simulink model "bh_slopey_floor_rolling_sphere_MASK"  (R2020b)
settings: Solver=ode15s  StartTime=0.0  StopTime=6  FixedStep=0.001  RelTol=1e-6  EnableMultiTasking=on
undefined symbols (not defined in the file): X, Y, Z
libraries: nesl_utility x25, sm_lib x21
settings Model: EnablePacing=on  Creator=scastro  LastModifiedBy=bhorton
settings SolverCC: ZeroCrossAlgorithm=Adaptive
settings DataIOCC: LimitDataPoints=on  ReturnWorkspaceOutputs=off
settings OptimizationCC: BlockReduction=off  LifeSpan=inf
settings DebuggingCC: AllowSymbolicDim=off  SFUnexpectedBacktrackingDiag=warning  SFNoUnconditionalDefaultTransitionDiag=warning  SFExecutionAtInitializationDiag=none  ArithmeticOperatorsInVariantConditions=warning
settings SFSimCC: SimUseLocalCustomCode=off  CustomCodeUndefinedFunction=UseInterfaceOnly
settings RTWCC: RTWUseLocalCustomCode=off
settings CodeAppCC: StateflowObjectComments=on
settings GRTTargetCC: TargetLangStandard=C89/C90 (ANSI)
settings ConfigComp: CovMetricSettings=dw  CovSaveCumulativeToWorkspaceVar=on  CovSaveSingleToWorkspaceVar=on  CovExternalEMLEnable=off  CovSFcnEnable=off
settings SimscapeCC: SimscapeNormalizeSystem=off  SimscapeLogType=all  SimscapeLogLimitData=off  SimscapeLogDataHistory=10000
settings ConfigurationSet: Description=SimMechanics 2G
settings DiagnosticsConfigSet: SimMechanicsRigidlyBoundBlock=none
settings ExplorerConfigSet: InternalSimMechanicsExplorerSettings="<ExplorerConfiguration><canonicalview>default</canonicalview><AnimationSetting><BasePlaybackSpeed>1.0</BasePlaybackSpeed><PlaybackSpeedFactor>1.0</PlaybackSpeedFactor></AnimationSetting><TilePanel><TileInfo><Tiles Columns=\"2\" Count=\"4\" Rows=\"2\"><Column Weight=\"0.4996\"/><Column Weight=\"0.5004\"/><Row Weight=\"0.4994\"/><Row Weight=\"0.5006\"/><Tile Height=\"1\" Width=\"1\" X=\"0\" Y=\"0\"/><Tile Height=\"1\" Width=\"1\" X=\"0\" Y=\"1\"/><Tile Height=\"1\" Width=\"1\" X=\"1\" Y=\"0\"/><Tile Height=\"1\" Width=\"1\" X=\"1\" Y=\"1\"/></Tiles></TileInfo><SceneInfo><SceneViewer><BGColor><R>0.60000002384185791</R><G>0.60000002384185791</G><B>0.60000002384185791</B></BGColor><Camera><DoPerspective>off</DoPerspective><Position><X>2.25966727667424827</X><Y>-62.0130897867078019</Y><Z>-2.35818613645341157</Z></Position><Center><X>2.25966727667424827</X><Y>-2.62125395139589656e-07</Y><Z>-2.35818613645341157</Z></Center><Up><X>0</X><Y>-0</Y><Z>1</Z></Up><ViewLimDist>1</ViewLimDist><YLim>12.1061815480941526</YLim><XLim>17.886610575562532</XLim></Camera></SceneViewer><SceneViewer><BGColor><R>0.60000002384185791</R><G>0.60000002384185791</G><B>0.60000002384185791</B></BGColor><Camera><DoPerspective>off</DoPerspective><Position><X>13.7336956207032639</X><Y>-7.76347886559767453</Y><Z>61.1905876504773261</Z></Position><Center><X>13.7336956207032639</X><Y>-7.76347886559767453</Y><Z>-0.181522868139726512</Z></Center><Up><X>0</X><Y>1</Y><Z>-0</Z></Up><ViewLimDist>1</ViewLimDist><YLim>19.5392058706914682</YLim><XLim>28.7392803837973183</XLim></Camera></SceneViewer><SceneViewer><BGColor><R>0.60000002384185791</R><G>0.60000002384185791</G><B>0.60000002384185791</B></BGColor><Camera><DoPerspective>off</DoPerspective><Position><X>62.80059271421446</X><Y>5.74913462249758478</Y><Z>-9.58222127968170945</Z></Position><Center><X>1.37359199311038616</X><Y>5.74913462249758478</Y><Z>-9.58222127968170945</Z></Center><Up><X>-0</X><Y>0</Y><Z>1</Z></Up><ViewLimDist>1</ViewLimDist><YLim>22.3277388712980738</YLim><XLim>33.0893067056624588</XLim></Camera></SceneViewer><SceneViewer><BGColor><R>0.60000002384185791</R><G>0.60000002384185791</G><B>0.60000002384185791</B></BGColor><Camera><DoPerspective>off</DoPerspective><Position><X>61.5862213655142483</X><Y>-21.6336600450757075</Y><Z>3.54423065630081169</Z></Position><Center><X>22.1204892369751072</X><Y>14.8464342674815555</Y><Z>-10.516698059065412</Z></Center><Up><X>-0.213092164247365046</X><Y>0.142054424815019287</Y><Z>0.9666500245315508</Z></Up><ViewLimDist>1</ViewLimDist><YLim>31.0369134821928654</YLim><XLim>45.7898858100513593</XLim></Camera></SceneViewer></SceneInfo></TilePanel><MechEditorPanel><Cameras/><GfxPanelCameraMap/><VideoCreator><PlaybackSpeedRatio>1.0</PlaybackSpeedRatio><FrameRate>30</FrameRate><VideoFormat>Motion JPEG AVI</VideoFormat><FrameSize>auto</FrameSize></VideoCreator></MechEditorPanel></ExplorerConfiguration>"

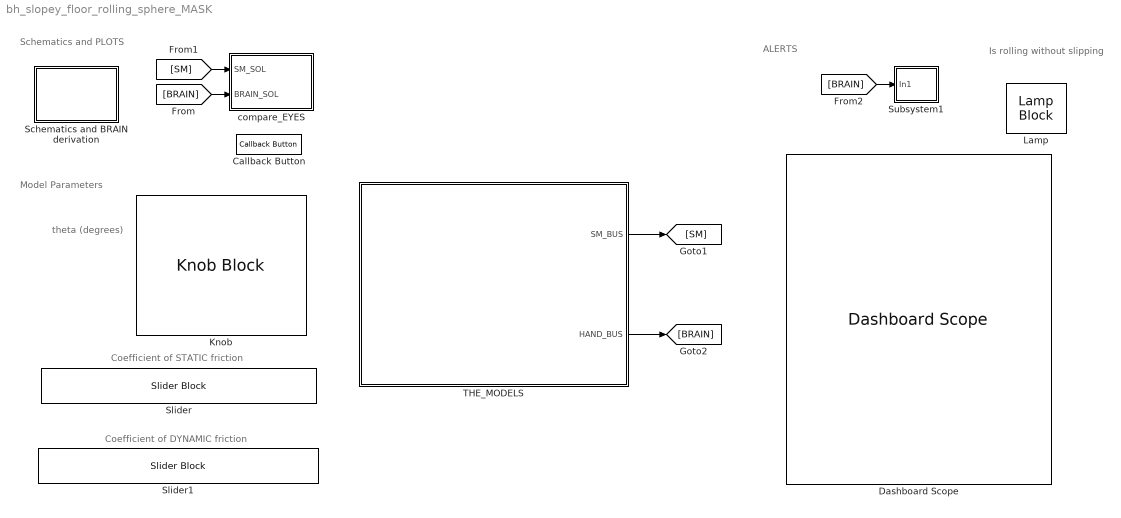
== system bh_slopey_floor_rolling_sphere_MASK ==
  note: Is rolling without slipping
  note: ALERTS
  note: theta (degrees)
  note: Model Parameters
  note: Schematics and PLOTS
  note: Coefficient of DYNAMIC friction
  note: Coefficient of STATIC friction
  Callback Button : CallbackButton  ButtonText=OPEN scope
      settings: ClickFcn="open_system(bdroot+\"/compare_EYES/compare_scope\")"
  Dashboard Scope : DashboardScope
  Knob : KnobBlock  LabelPosition=Hide  ScaleMin=5  ScaleMax=75  TickInterval=5
  Lamp : LampBlock
  Schematics and BRAIN derivation : Subsystem
  Slider : SliderBlock  LabelPosition=Hide  ScaleMax=0.5  TickInterval=0.05
  Slider1 : SliderBlock  LabelPosition=Hide  ScaleMax=0.3  TickInterval=0.05
  Subsystem1 : Subsystem
  THE_MODELS : Subsystem  mask{sphRad=1.5, sphMass=1, theta_deg=30, mu_static=0.5, mu_dynamic=0.3, g=9.80665}
      mask prompts: sphRad "Radius  (m)"; sphMass "Mass (kg)"; theta_deg "theta  (DEGREES)"; mu_static "Coefficient of STATIC friction"; mu_dynamic "Coefficient of DYNAMIC friction"; g "g  (m/sec^2)"
      mask DialogControl Container4 Prompt: Sphere
      mask DialogControl Container5 Prompt: Floor
      mask DialogControl Container6 Prompt: Friction
      mask DialogControl Container7 Prompt: Environment
      mask Display: image('bh_MASK_PIC_DO_NOT_DELETE.PNG'); % Use "Edit Image" on toolstrip to change.
  compare_EYES : Subsystem
  wires:
  [SM] -> compare_EYES/1(SM_SOL)
  [BRAIN] -> compare_EYES/2(BRAIN_SOL)
  THE_MODELS/1(SM_BUS) -> [SM]
  THE_MODELS/2(HAND_BUS) -> [BRAIN]
  [BRAIN] -> Subsystem1/1(In1)

== system bh_slopey_floor_rolling_sphere_MASK/Schematics and BRAIN derivation ==
  note: Open the BRAIN derivation
  note: Open the Simulink implementation of the BRAIN derivation
  Callback Button : CallbackButton  ButtonText=Open the BRAIN Derivation
      settings: ClickFcn=open bh_hand_deriv_sphere_on_slopey_floor.PDF
  Callback Button1 : CallbackButton  ButtonText=Open the Simulink Implementation
      settings: ClickFcn=|
      | THE_SYS = [bdroot,'/THE_MODELS/BRAIN_SOLUTION'];
      | open_system(THE_SYS)

== system bh_slopey_floor_rolling_sphere_MASK/Subsystem1 ==
  In1 : Inport
  Bus Selector : BusSelector  OutputSignals=tf_is_rolling,Ff_mag,N,muStat_times_N
  Terminator{,1..3} (4 alike) : Terminator
  wires:
  In1/1 -> Bus Selector/1
  Bus Selector/1 -> Terminator/1  "<tf_is_rolling>"
  Bus Selector/2 -> Terminator1/1  "<Ff_mag>"
  Bus Selector/3 -> Terminator2/1  "<N>"
  Bus Selector/4 -> Terminator3/1  "<muStat_times_N>"

== system bh_slopey_floor_rolling_sphere_MASK/THE_MODELS ==
  BRAIN_SOLUTION : Subsystem
  Simscape_Model : Subsystem
  SM_BUS : Outport
  HAND_BUS : Outport  Port=2
  wires:
  Simscape_Model/1(SM_BUS) -> SM_BUS/1
  BRAIN_SOLUTION/1(HAND_SOL) -> HAND_BUS/1

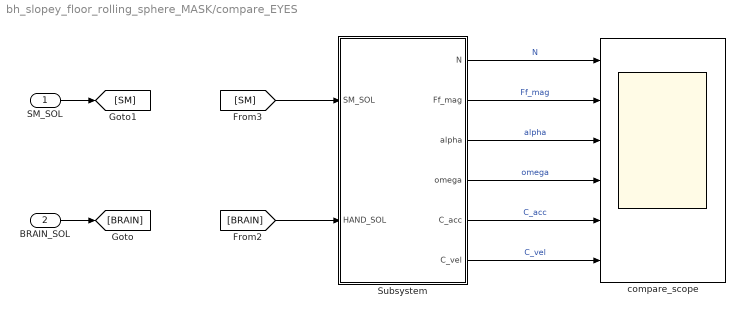
== system bh_slopey_floor_rolling_sphere_MASK/compare_EYES ==
  SM_SOL : Inport
  BRAIN_SOL : Inport  Port=2
  Subsystem : Subsystem
  compare_scope : Scope  NumInputPorts=6
  wires:
  BRAIN_SOL/1 -> [BRAIN]
  SM_SOL/1 -> [SM]
  [BRAIN] -> Subsystem/2(HAND_SOL)
  [SM] -> Subsystem/1(SM_SOL)
  Subsystem/1(N) -> compare_scope/1  "N"
  Subsystem/2(Ff_mag) -> compare_scope/2  "Ff_mag"
  Subsystem/3(alpha) -> compare_scope/3  "alpha"
  Subsystem/4(omega) -> compare_scope/4  "omega"
  Subsystem/5(C_acc) -> compare_scope/5  "C_acc"
  Subsystem/6(C_vel) -> compare_scope/6  "C_vel"

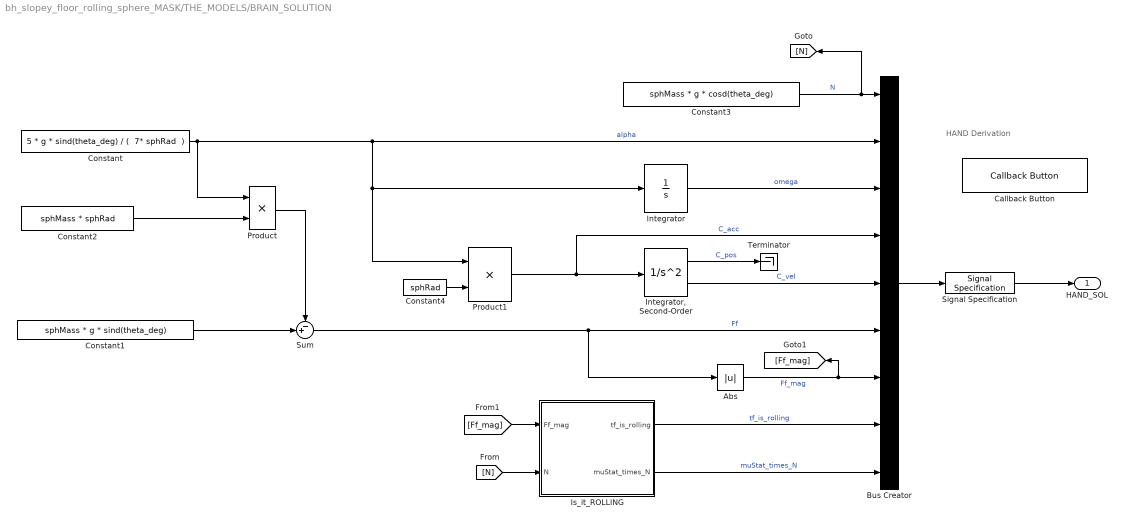
== system bh_slopey_floor_rolling_sphere_MASK/THE_MODELS/BRAIN_SOLUTION ==
  note: HAND Derivation
  Abs : Abs
  Bus Creator : BusCreator  Inputs=9
  Callback Button : CallbackButton  ButtonText=Open the hand Derivation
      settings: ClickFcn=open bh_hand_deriv_sphere_on_slopey_floor.PDF
  Constant : Constant  Value="5 * g * sind(theta_deg) / (  7* sphRad  )"
  Constant1 : Constant  Value=sphMass * g * sind(theta_deg)
  Constant2 : Constant  Value=sphMass * sphRad
  Constant3 : Constant  Value=sphMass * g * cosd(theta_deg)
  Constant4 : Constant  Value=sphRad
  Integrator : Integrator
  "Integrator, Second-Order" : SecondOrderIntegrator
  Is_it_ROLLING : Subsystem
  Product : Product
  Product1 : Product
  Signal Specification : SignalSpecification  SampleTime=0
  Sum : Sum  Inputs=-+|
  Terminator : Terminator
  HAND_SOL : Outport
  wires:
  Constant/1 -> Bus Creator/2, Integrator/1, Product1/1, Product/1  "alpha"
  Constant2/1 -> Product/2
  Product/1 -> Sum/1
  Constant1/1 -> Sum/2
  Constant3/1 -> [N], Bus Creator/1  "N"
  Sum/1 -> Abs/1, Bus Creator/6  "Ff"
  Abs/1 -> [Ff_mag], Bus Creator/7  "Ff_mag"
  Integrator/1 -> Bus Creator/3  "omega"
  Product1/1 -> "Integrator, Second-Order"/1, Bus Creator/4  "C_acc"
  Constant4/1 -> Product1/2
  "Integrator, Second-Order"/1 -> Terminator/1  "C_pos"
  "Integrator, Second-Order"/2 -> Bus Creator/5  "C_vel"
  Bus Creator/1 -> Signal Specification/1
  Signal Specification/1 -> HAND_SOL/1
  [Ff_mag] -> Is_it_ROLLING/1(Ff_mag)
  [N] -> Is_it_ROLLING/2(N)
  Is_it_ROLLING/1(tf_is_rolling) -> Bus Creator/8  "tf_is_rolling"
  Is_it_ROLLING/2(muStat_times_N) -> Bus Creator/9  "muStat_times_N"

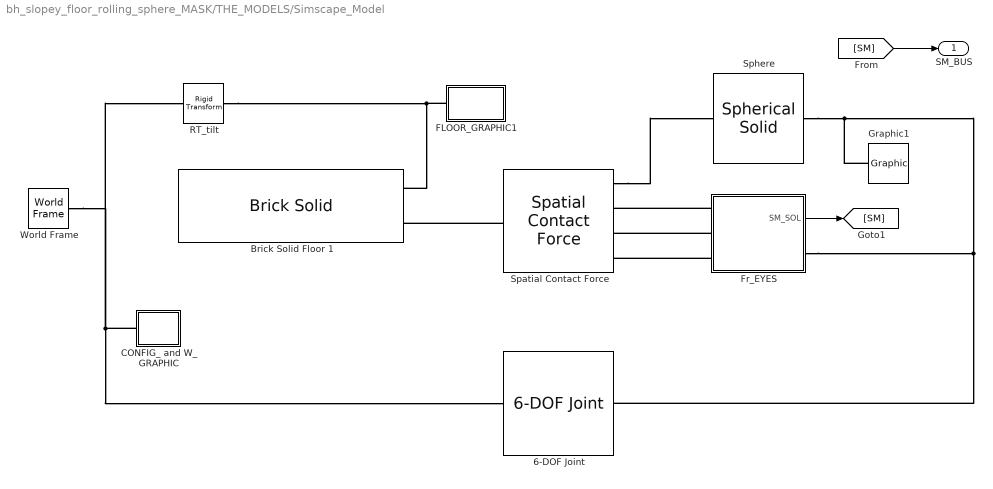
== system bh_slopey_floor_rolling_sphere_MASK/THE_MODELS/Simscape_Model ==
  6-DOF Joint : sm_lib/Joints/6-DOF Joint  JointMode=Normal  SenseConstraintForce=off  SenseConstraintForceX=off  SenseConstraintForceY=off  SenseConstraintForceZ=off  SenseConstraintTorque=off  SenseConstraintTorqueX=off  SenseConstraintTorqueY=off  SenseConstraintTorqueZ=off  SenseTotalForce=off  SenseTotalForceX=off  SenseTotalForceY=off  SenseTotalForceZ=off  SenseTotalTorque=off  SenseTotalTorqueX=off  SenseTotalTorqueY=off  SenseTotalTorqueZ=off  CompositeWrenchDir=FollowerOnBase  CompositeWrenchFrame=BaseFrame  PxEquilibriumPosition=0  PxEquilibriumPositionUnits=m  PxSpringStiffness=0  PxSpringStiffnessUnits=N/m  PxDampingCoefficient=0  PxDampingCoefficientUnits=N/(m/s)  PxTorqueActuationMode=NoTorque  PxMotionActuationMode=ComputedMotion  PxSensePosition=off  PxSenseVelocity=off  PxSenseAcceleration=off  PxSenseTorqueForce=off  PxSenseLowerLimitTorqueForce=off  PxSenseUpperLimitTorqueForce=off  PxLowerLimitSpecify=off  PxLowerLimitBound=-1  PxLowerLimitBoundUnits=m  PxLowerLimitStiffness=1e6  PxLowerLimitStiffnessUnits=N/m  PxLowerLimitDamping=1e3  PxLowerLimitDampingUnits=N/(m/s)  PxLowerLimitTransitionRegionWidth=1e-4  PxLowerLimitTransitionRegionWidthUnits=m  PxUpperLimitSpecify=off  PxUpperLimitBound=1  PxUpperLimitBoundUnits=m  PxUpperLimitStiffness=1e6  PxUpperLimitStiffnessUnits=N/m  PxUpperLimitDamping=1e3  PxUpperLimitDampingUnits=N/(m/s)  PxUpperLimitTransitionRegionWidth=1e-4  PxUpperLimitTransitionRegionWidthUnits=m  PxPositionTargetSpecify=on  PxPositionTargetPriority=High  PxPositionTargetValue=sphRad*sind(theta_deg)  PxPositionTargetValueUnits=m  PxVelocityTargetSpecify=off  PxVelocityTargetPriority=High  PxVelocityTargetValue=0  PxVelocityTargetValueUnits=m/s  PyEquilibriumPosition=0  PyEquilibriumPositionUnits=m  PySpringStiffness=0  PySpringStiffnessUnits=N/m  PyDampingCoefficient=0  PyDampingCoefficientUnits=N/(m/s)  PyTorqueActuationMode=NoTorque  PyMotionActuationMode=ComputedMotion  PySensePosition=off  PySenseVelocity=off  PySenseAcceleration=off  PySenseTorqueForce=off  PySenseLowerLimitTorqueForce=off  PySenseUpperLimitTorqueForce=off  PyLowerLimitSpecify=off  PyLowerLimitBound=-1  PyLowerLimitBoundUnits=m  PyLowerLimitStiffness=1e6  PyLowerLimitStiffnessUnits=N/m  PyLowerLimitDamping=1e3  PyLowerLimitDampingUnits=N/(m/s)  PyLowerLimitTransitionRegionWidth=1e-4  PyLowerLimitTransitionRegionWidthUnits=m  PyUpperLimitSpecify=off  PyUpperLimitBound=1  PyUpperLimitBoundUnits=m  PyUpperLimitStiffness=1e6  PyUpperLimitStiffnessUnits=N/m  PyUpperLimitDamping=1e3  PyUpperLimitDampingUnits=N/(m/s)  PyUpperLimitTransitionRegionWidth=1e-4  PyUpperLimitTransitionRegionWidthUnits=m  PyPositionTargetSpecify=on  PyPositionTargetPriority=High  PyPositionTargetValue=0  PyPositionTargetValueUnits=m  PyVelocityTargetSpecify=off  PyVelocityTargetPriority=High  PyVelocityTargetValue=0  PyVelocityTargetValueUnits=m/s  PzEquilibriumPosition=0  PzEquilibriumPositionUnits=m  PzSpringStiffness=0  PzSpringStiffnessUnits=N/m  PzDampingCoefficient=0  PzDampingCoefficientUnits=N/(m/s)  PzTorqueActuationMode=NoTorque  PzMotionActuationMode=ComputedMotion  PzSensePosition=off  PzSenseVelocity=off  PzSenseAcceleration=off  PzSenseTorqueForce=off  PzSenseLowerLimitTorqueForce=off  PzSenseUpperLimitTorqueForce=off  PzLowerLimitSpecify=off  PzLowerLimitBound=-1  PzLowerLimitBoundUnits=m  PzLowerLimitStiffness=1e6  PzLowerLimitStiffnessUnits=N/m  PzLowerLimitDamping=1e3  PzLowerLimitDampingUnits=N/(m/s)  PzLowerLimitTransitionRegionWidth=1e-4  PzLowerLimitTransitionRegionWidthUnits=m  PzUpperLimitSpecify=off  PzUpperLimitBound=1  PzUpperLimitBoundUnits=m  PzUpperLimitStiffness=1e6  PzUpperLimitStiffnessUnits=N/m  PzUpperLimitDamping=1e3  PzUpperLimitDampingUnits=N/(m/s)  PzUpperLimitTransitionRegionWidth=1e-4  PzUpperLimitTransitionRegionWidthUnits=m  PzPositionTargetSpecify=on  PzPositionTargetPriority=High  PzPositionTargetValue=sphRad*cosd(theta_deg)  PzPositionTargetValueUnits=m  PzVelocityTargetSpecify=off  PzVelocityTargetPriority=High  PzVelocityTargetValue=0  PzVelocityTargetValueUnits=m/s  SphDefPosRotationMethod=None  SphDefPosRotationAngleUnits=deg  SphDefPosRotationStandardAxis=+Z  SphDefPosRotationAngle=0.0  SphDefPosRotationArbitraryAxis=[0 0 1]  SphDefPosFollAlignAxisA=+X  SphDefPosBaseAlignAxisA=+Y  SphDefPosFollAlignAxisB=+Y  SphDefPosBaseAlignAxisB=+Z  SphDefPosRotationSequenceAxes=FollowerAxes  SphDefPosRotationSequence=XYX  SphDefPosRotationSequenceAngles=[0 0 0]  SphDefPosRotationSequenceAnglesUnits=deg  SphDefPosRotationMatrix=[1 0 0; 0 1 0; 0 0 1]  SphEqPosRotationMethod=None  SphEqPosRotationAngleUnits=deg  SphEqPosRotationStandardAxis=+Z  SphEqPosRotationAngle=0.0  SphEqPosRotationArbitraryAxis=[0 0 1]  SphEqPosFollAlignAxisA=+X  SphEqPosBaseAlignAxisA=+Y  SphEqPosFollAlignAxisB=+Y  SphEqPosBaseAlignAxisB=+Z  SphEqPosRotationSequenceAxes=FollowerAxes  SphEqPosRotationSequence=XYX  SphEqPosRotationSequenceAngles=[0 0 0]  SphEqPosRotationSequenceAnglesUnits=deg  SphEqPosRotationMatrix=[1 0 0; 0 1 0; 0 0 1]  SphSpringStiffness=0  SphSpringStiffnessUnits=N*m/deg  SphDampingCoefficient=0  SphDampingCoefficientUnits=N*m/(deg/s)  SphActuateTorqueX=off  SphActuateTorqueY=off  SphActuateTorqueZ=off  SphActuateTorque=off  SphTorqueActuationMode=NoTorque  SphMotionActuationMode=ComputedMotion  SphActuationFrame=BaseFrame  SphSensePosition=off  SphSenseVelocityX=off  SphSenseVelocityY=off  SphSenseVelocityZ=off  SphSenseVelocity=off  SphSenseAccelerationX=off  SphSenseAccelerationY=off  SphSenseAccelerationZ=off  SphSenseAcceleration=off  SphSenseTorqueX=off  SphSenseTorqueY=off  SphSenseTorqueZ=off  SphSenseTorqueForce=off  SphSenseLowerLimitTorqueMag=off  SphSenseUpperLimitTorqueMag=off  SphSensingFrame=BaseFrame  SphLowerLimitSpecify=off  SphLowerLimitBound=15  SphLowerLimitBoundUnits=deg  SphLowerLimitStiffness=1e4  SphLowerLimitStiffnessUnits=N*m/deg  SphLowerLimitDamping=10  SphLowerLimitDampingUnits=N*m/(deg/s)  SphLowerLimitTransitionRegionWidth=0.1  SphLowerLimitTransitionRegionWidthUnits=deg  SphUpperLimitSpecify=off  SphUpperLimitBound=45  SphUpperLimitBoundUnits=deg  SphUpperLimitStiffness=1e4  SphUpperLimitStiffnessUnits=N*m/deg  SphUpperLimitDamping=10  SphUpperLimitDampingUnits=N*m/(deg/s)  SphUpperLimitTransitionRegionWidth=0.1  SphUpperLimitTransitionRegionWidthUnits=deg  SphPositionTargetRotationMethod=None  SphPositionTargetRotationAngleUnits=deg  SphPositionTargetRotationStandardAxis=+Z  SphPositionTargetRotationAngle=0.0  SphPositionTargetRotationArbitraryAxis=[0 0 1]  SphPositionTargetFollAlignAxisA=+X  SphPositionTargetBaseAlignAxisA=+Y  SphPositionTargetFollAlignAxisB=+Y  SphPositionTargetBaseAlignAxisB=+Z  SphPositionTargetRotationSequenceAxes=FollowerAxes  SphPositionTargetRotationSequence=XYX  SphPositionTargetRotationSequenceAngles=[0 0 0]  SphPositionTargetRotationSequenceAnglesUnits=deg  SphPositionTargetRotationMatrix=[1 0 0; 0 1 0; 0 0 1]  SphPositionTargetSpecify=on  SphPositionTargetPriority=High  SphVelocityTargetValue=[0 0 0]  SphVelocityTargetValueUnits=deg/s  SphVelocityTargetSpecify=off  SphVelocityTargetPriority=High  SphVelocityTargetInFollowerFrame=on
      settings: AttributesFormatString=IC_POS = [ %<PxPositionTargetValue> , %<PyPositionTargetValue> , %<PzPositionTargetValue> ]
  Brick Solid Floor 1 : sm_lib/Body Elements/Brick Solid  GraphicAmbientColor=[0.15 0.15 0.15 1.0]  BasedOnType=Density  BrickDimensions=[100,10,2]  BrickDimensionUnits=m  CenterOfMass=[0 0 0]  CenterOfMassUnits=m  GraphicDiffuseColor=[1.0 1.0 0.4]  Density=1000  DensityUnits=kg/m^3  DoExposeReferenceFrame=on  GraphicEmissiveColor=[0.0 0.0 0.0 1.0]  ExportEntireGeometry=on  SerializedFrames=<Frames><Frame><Id>Frame1</Id><Value><Name>F</Name><Origin><Source>GeometricFeature</Source><FeatureName>+z surface</FeatureName></Origin><PrimaryAxis><DefinedDirection>+Z</DefinedDirection><Source>ReferenceFrame</Source><SourceDirection>+Z</SourceDirection><FeatureName></FeatureName></PrimaryAxis><SecondaryAxis><DefinedDirection>+X</DefinedDirection><Source>ReferenceFrame</Source><SourceDirection>+X</SourceDirection><FeatureName></FeatureName></SecondaryAxis></Value></Frame></Frames>  MarkerShape=Sphere  MarkerSize=10  GraphicType=FromGeometry  InertiaType=CalculateFromGeometry  Mass=1  MassUnits=kg  MomentsOfInertia=[1 1 1]  MomentsOfInertiaUnits=kg*m^2  GraphicOpacity=1.0  ProductsOfInertia=[0 0 0]  ProductsOfInertiaUnits=kg*m^2  GraphicShininess=75  GraphicSpecularColor=[0.5 0.5 0.5 1.0]  GraphicVisPropType=SimpleVisualProperties
      settings: AttributesFormatString=Size: %<BrickDimensions>
  CONFIG_ and W_GRAPHIC : Subsystem
  FLOOR_GRAPHIC1 : Subsystem
  Fr_EYES : Subsystem
  Graphic1 : sm_lib/Body Elements/Graphic  GraphicType=Marker  MarkerShape=Frame  MarkerSize=45  GraphicVisPropType=SimpleVisualProperties  GraphicDiffuseColor=[1.0 0.0 0.2]  GraphicSpecularColor=[0.5 0.5 0.5 1.0]  GraphicAmbientColor=[0.15 0.15 0.15 1.0]  GraphicEmissiveColor=[0.0 0.0 0.0 1.0]  GraphicShininess=75  GraphicOpacity=1.0
  RT_tilt : sm_lib/Frames and Transforms/Rigid Transform  TranslationMethod=None  TranslationStandardOffset=0  TranslationLengthUnit=m  TranslationStandardAxis=+Z  TranslationCartesianOffset=[0 0 0]  TranslationROffset=0  TranslationROffsetUnits=m  TranslationZOffset=0  TranslationZOffsetUnits=m  TranslationThetaOffset=0  TranslationThetaOffsetUnits=deg  RotationMethod=StandardAxis  RotationAngleUnits=deg  RotationStandardAxis=+Y  RotationAngle=theta_deg  RotationArbitraryAxis=[0 0 1]  FollAlignAxisA=+X  BaseAlignAxisA=+Y  FollAlignAxisB=+Y  BaseAlignAxisB=+Z  RotationSequenceAxes=FollowerAxes  RotationSequence=XYX  RotationSequenceAngles=[0 0 0]  RotationSequenceAnglesUnits=deg  RotationMatrix=[1 0 0; 0 1 0; 0 0 1]
  Spatial Contact Force : sm_lib/Forces and Torques/Spatial Contact Force  CoefficientOfDynamicFriction=mu_dynamic  CoefficientOfStaticFriction=mu_static  NormalDamping=5e4  NormalDampingUnits=N/(m/s)  NormalStiffness=1e6  NormalStiffnessUnits=N/m  FrictionalCriticalVelocity=5e-3  FrictionalCriticalVelocityUnits=m/s  ZeroCrossDetectContactStartAndEnd=on  SenseFrictionalForceMagnitude=on  SenseNormalForceMagnitude=on  SenseSeparationDistance=on  NormalTransitionRegionWidth=1e-4  NormalTransitionRegionWidthUnits=m  FrictionType=SmoothStickSlip
  Sphere : sm_lib/Body Elements/Spherical Solid  GraphicAmbientColor=[0.15 0.15 0.15 1.0]  BasedOnType=Mass  CenterOfMass=[0 0 0]  CenterOfMassUnits=m  GraphicDiffuseColor=[1.0 0.0 0.2]  Density=1000  DensityUnits=kg/m^3  DoExposeReferenceFrame=on  GraphicEmissiveColor=[0.0 0.0 0.0 1.0]  ExportEntireGeometry=on  SerializedExposedGeometries=<ExposedGeometries><ExposedGeometry><RawGeometryId>entire</RawGeometryId><ExposedGeometryId>G</ExposedGeometryId></ExposedGeometry></ExposedGeometries>  SerializedFrames=<Frames/>  MarkerShape=Sphere  MarkerSize=10  GraphicType=FromGeometry  InertiaType=CalculateFromGeometry  Mass=sphMass  MassUnits=kg  MomentsOfInertia=[1 1 1]  MomentsOfInertiaUnits=kg*m^2  GraphicOpacity=1.0  ProductsOfInertia=[1 1 1]  ProductsOfInertiaUnits=kg*m^2  GraphicShininess=75  GraphicSpecularColor=[0.5 0.5 0.5 1.0]  SphereRadius=sphRad  SphereRadiusUnits=m  GraphicVisPropType=SimpleVisualProperties
      settings: AttributesFormatString=|
      | Radius = %<SphereRadius>
      | Mass = %<Mass>
  World Frame : sm_lib/Frames and Transforms/World Frame
  SM_BUS : Outport
  wires:
  Fr_EYES/1(SM_SOL) -> [SM]
  [SM] -> SM_BUS/1
  connections:
  Fr_EYES/LConn3 -- Spatial Contact Force/RConn4
  RT_tilt/LConn1 -- World Frame/RConn1 -- 6-DOF Joint/LConn1 -- CONFIG_ and W_GRAPHIC/LConn1
  Fr_EYES/LConn2 -- Spatial Contact Force/RConn3
  Fr_EYES/LConn1 -- Spatial Contact Force/RConn2
  RT_tilt/RConn1 -- FLOOR_GRAPHIC1/LConn1 -- Brick Solid Floor 1/LConn1
  Sphere/RConn1 -- Fr_EYES/RConn1 -- 6-DOF Joint/RConn1 -- Graphic1/RConn1
  Spatial Contact Force/RConn1 -- Sphere/LConn1
  Spatial Contact Force/LConn1 -- Brick Solid Floor 1/LConn2

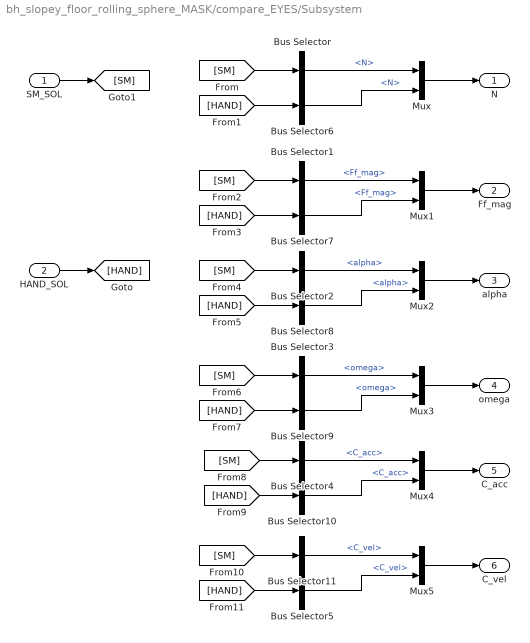
== system bh_slopey_floor_rolling_sphere_MASK/compare_EYES/Subsystem ==
  SM_SOL : Inport
  HAND_SOL : Inport  Port=2
  Bus Selector : BusSelector  OutputSignals=N
  Bus Selector1 : BusSelector  OutputSignals=Ff_mag
  Bus Selector10 : BusSelector  OutputSignals=C_acc
  Bus Selector11 : BusSelector  OutputSignals=C_vel
  Bus Selector2 : BusSelector  OutputSignals=alpha
  Bus Selector3 : BusSelector  OutputSignals=omega
  Bus Selector4 : BusSelector  OutputSignals=C_acc
  Bus Selector5 : BusSelector  OutputSignals=C_vel
  Bus Selector6 : BusSelector  OutputSignals=N
  Bus Selector7 : BusSelector  OutputSignals=Ff_mag
  Bus Selector8 : BusSelector  OutputSignals=alpha
  Bus Selector9 : BusSelector  OutputSignals=omega
  Mux{,1..5} (6 alike) : Mux  Inputs=2
  N : Outport
  Ff_mag : Outport  Port=2
  alpha : Outport  Port=3
  omega : Outport  Port=4
  C_acc : Outport  Port=5
  C_vel : Outport  Port=6
  wires:
  Mux/1 -> N/1
  HAND_SOL/1 -> [HAND]
  SM_SOL/1 -> [SM]
  Bus Selector/1 -> Mux/1  "<N>"
  [SM] -> Bus Selector/1
  [HAND] -> Bus Selector6/1
  Mux1/1 -> Ff_mag/1
  Bus Selector1/1 -> Mux1/1  "<Ff_mag>"
  [HAND] -> Bus Selector7/1
  [SM] -> Bus Selector1/1
  [HAND] -> Bus Selector8/1
  [SM] -> Bus Selector2/1
  [HAND] -> Bus Selector9/1
  [SM] -> Bus Selector3/1
  [HAND] -> Bus Selector10/1
  [SM] -> Bus Selector4/1
  [HAND] -> Bus Selector5/1
  [SM] -> Bus Selector11/1
  Bus Selector6/1 -> Mux/2  "<N>"
  Bus Selector7/1 -> Mux1/2  "<Ff_mag>"
  Mux2/1 -> alpha/1
  Bus Selector2/1 -> Mux2/1  "<alpha>"
  Bus Selector8/1 -> Mux2/2  "<alpha>"
  Mux3/1 -> omega/1
  Bus Selector3/1 -> Mux3/1  "<omega>"
  Bus Selector9/1 -> Mux3/2  "<omega>"
  Mux4/1 -> C_acc/1
  Bus Selector4/1 -> Mux4/1  "<C_acc>"
  Bus Selector10/1 -> Mux4/2  "<C_acc>"
  Mux5/1 -> C_vel/1
  Bus Selector11/1 -> Mux5/1  "<C_vel>"
  Bus Selector5/1 -> Mux5/2  "<C_vel>"

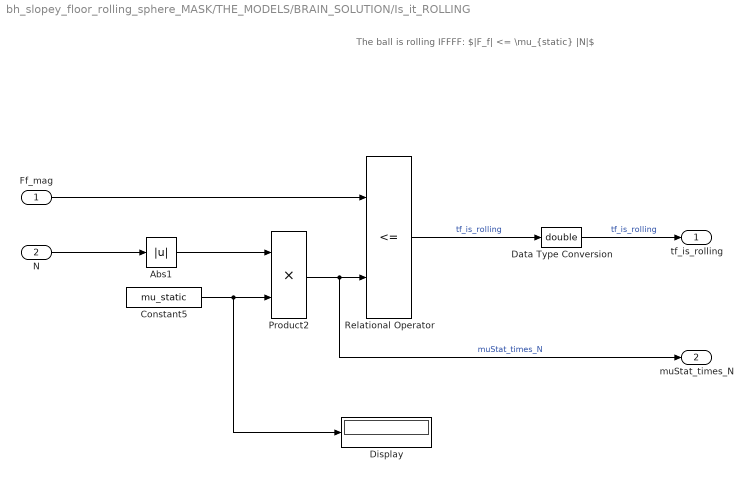
== system bh_slopey_floor_rolling_sphere_MASK/THE_MODELS/BRAIN_SOLUTION/Is_it_ROLLING ==
  note: The ball is rolling IFFFF:
      |
      | $|F_f| <= \mu_{static} |N|$
  Ff_mag : Inport
  N : Inport  Port=2
  Abs1 : Abs
  Constant5 : Constant  Value=mu_static
  Data Type Conversion : DataTypeConversion  OutDataTypeStr=double
  Display : Display
  Product2 : Product
  Relational Operator : RelationalOperator  Operator=<=  OutDataTypeStr=boolean  RndMeth=Simplest
  tf_is_rolling : Outport
  muStat_times_N : Outport  Port=2
  wires:
  Ff_mag/1 -> Relational Operator/1
  Product2/1 -> muStat_times_N/1, Relational Operator/2  "muStat_times_N"
  N/1 -> Abs1/1
  Relational Operator/1 -> Data Type Conversion/1  "tf_is_rolling"
  Abs1/1 -> Product2/1
  Constant5/1 -> Display/1, Product2/2
  Data Type Conversion/1 -> tf_is_rolling/1  "tf_is_rolling"

== system bh_slopey_floor_rolling_sphere_MASK/THE_MODELS/Simscape_Model/CONFIG_ and W_GRAPHIC ==
  Graphic : sm_lib/Body Elements/Graphic  GraphicType=Marker  MarkerShape=Frame  MarkerSize=45  GraphicVisPropType=SimpleVisualProperties  GraphicDiffuseColor=[0.0 0.0 0.0]  GraphicSpecularColor=[0.5 0.5 0.5 1.0]  GraphicAmbientColor=[0.15 0.15 0.15 1.0]  GraphicEmissiveColor=[0.0 0.0 0.0 1.0]  GraphicShininess=75  GraphicOpacity=1.0
  Mechanism Configuration : sm_lib/Utilities/Mechanism Configuration  UniformGravity=Constant  GravityVector=[0 0 -g]  GravityVectorUnits=m/s^2  GravityUnits=m/s^2  LinearizationDelta=0.001  JointModeTransitionNonlinearIterations=2
  Rigid Transform : sm_lib/Frames and Transforms/Rigid Transform  TranslationMethod=StandardAxis  TranslationStandardOffset=15  TranslationLengthUnit=m  TranslationStandardAxis=-X  TranslationCartesianOffset=[0 0 0]  TranslationROffset=0  TranslationROffsetUnits=m  TranslationZOffset=0  TranslationZOffsetUnits=m  TranslationThetaOffset=0  TranslationThetaOffsetUnits=deg  RotationMethod=None  RotationAngleUnits=deg  RotationStandardAxis=+Z  RotationAngle=0.0  RotationArbitraryAxis=[0 0 1]  FollAlignAxisA=+Y  BaseAlignAxisA=+Y  FollAlignAxisB=+Z  BaseAlignAxisB=+X  RotationSequenceAxes=FollowerAxes  RotationSequence=XYX  RotationSequenceAngles=[0 0 0]  RotationSequenceAnglesUnits=deg  RotationMatrix=[1 0 0; 0 1 0; 0 0 1]
  Rigid Transform1 : sm_lib/Frames and Transforms/Rigid Transform  TranslationMethod=StandardAxis  TranslationStandardOffset=15  TranslationLengthUnit=m  TranslationStandardAxis=-Y  TranslationCartesianOffset=[0 0 0]  TranslationROffset=0  TranslationROffsetUnits=m  TranslationZOffset=0  TranslationZOffsetUnits=m  TranslationThetaOffset=0  TranslationThetaOffsetUnits=deg  RotationMethod=None  RotationAngleUnits=deg  RotationStandardAxis=+Z  RotationAngle=0.0  RotationArbitraryAxis=[0 0 1]  FollAlignAxisA=+Y  BaseAlignAxisA=+Y  FollAlignAxisB=+Z  BaseAlignAxisB=+X  RotationSequenceAxes=FollowerAxes  RotationSequence=XYX  RotationSequenceAngles=[0 0 0]  RotationSequenceAnglesUnits=deg  RotationMatrix=[1 0 0; 0 1 0; 0 0 1]
  Solver Configuration : nesl_utility/Solver Configuration  PhysicalDomain=network_engine_domain  SubClassName=solver  LeftPortType=input  RightPortType=generic  Tones=[]  Harmonics=[]  SimulateNoise=off  Profile=off  UseLocalSampling=off  EnableSwitchedLinearOptims=on  FrequencyDomain=off  UseCCode=off  RelTol=0.001  AbsTol=1e-06  MinStep=1e-09  ToWorkspace=off  RevertToSquareIcSolve=off  NumHomotopyIterations=100  PhasorMode=off  PhasorModeNumHarmonics=1  DoDC=off  ResidualTolerance=1e-09  UseLocalSolver=off  LocalSolverChoice=NE_BACKWARD_EULER_ADVANCER  LocalSolverSampleTime=0.001  DoFixedCost=off  MaxNonlinIter=3  MaxModeIter=2  ComputeImpulses=off  ImpulseIterations=2  LinearAlgebra=Sparse  EquationFormulation=NE_TIME_EF  DelaysMemoryBudget=1024  AutomaticFiltering=on  FilteringTimeConstant=0.001  PartitionStorageMethod=AS_NEEDED  PartitionMemoryBudget=1024  PartitionMethod=FAST
  W : PMIOPort  Side=Left
  connections:
  W/RConn1 -- Mechanism Configuration/RConn1 -- Solver Configuration/RConn1 -- Rigid Transform/LConn1
  Rigid Transform1/RConn1 -- Graphic/RConn1
  Rigid Transform1/LConn1 -- Rigid Transform/RConn1

== system bh_slopey_floor_rolling_sphere_MASK/THE_MODELS/Simscape_Model/FLOOR_GRAPHIC1 ==
  Graphic : sm_lib/Body Elements/Graphic  GraphicType=Marker  MarkerShape=Frame  MarkerSize=45  GraphicVisPropType=SimpleVisualProperties  GraphicDiffuseColor=[0.0 0.0 1.0]  GraphicSpecularColor=[0.5 0.5 0.5 1.0]  GraphicAmbientColor=[0.15 0.15 0.15 1.0]  GraphicEmissiveColor=[0.0 0.0 0.0 1.0]  GraphicShininess=75  GraphicOpacity=1.0
  Rigid Transform : sm_lib/Frames and Transforms/Rigid Transform  TranslationMethod=StandardAxis  TranslationStandardOffset=15  TranslationLengthUnit=m  TranslationStandardAxis=-X  TranslationCartesianOffset=[0 0 0]  TranslationROffset=0  TranslationROffsetUnits=m  TranslationZOffset=0  TranslationZOffsetUnits=m  TranslationThetaOffset=0  TranslationThetaOffsetUnits=deg  RotationMethod=None  RotationAngleUnits=deg  RotationStandardAxis=+Z  RotationAngle=0.0  RotationArbitraryAxis=[0 0 1]  FollAlignAxisA=+Y  BaseAlignAxisA=+Y  FollAlignAxisB=+Z  BaseAlignAxisB=+X  RotationSequenceAxes=FollowerAxes  RotationSequence=XYX  RotationSequenceAngles=[0 0 0]  RotationSequenceAnglesUnits=deg  RotationMatrix=[1 0 0; 0 1 0; 0 0 1]
  Rigid Transform1 : sm_lib/Frames and Transforms/Rigid Transform  TranslationMethod=StandardAxis  TranslationStandardOffset=5  TranslationLengthUnit=m  TranslationStandardAxis=+Y  TranslationCartesianOffset=[0 0 0]  TranslationROffset=0  TranslationROffsetUnits=m  TranslationZOffset=0  TranslationZOffsetUnits=m  TranslationThetaOffset=0  TranslationThetaOffsetUnits=deg  RotationMethod=None  RotationAngleUnits=deg  RotationStandardAxis=+Z  RotationAngle=0.0  RotationArbitraryAxis=[0 0 1]  FollAlignAxisA=+Y  BaseAlignAxisA=+Y  FollAlignAxisB=+Z  BaseAlignAxisB=+X  RotationSequenceAxes=FollowerAxes  RotationSequence=XYX  RotationSequenceAngles=[0 0 0]  RotationSequenceAnglesUnits=deg  RotationMatrix=[1 0 0; 0 1 0; 0 0 1]
  FLOOR : PMIOPort  Side=Left
  connections:
  FLOOR/RConn1 -- Rigid Transform/LConn1
  Rigid Transform/RConn1 -- Rigid Transform1/LConn1
  Rigid Transform1/RConn1 -- Graphic/RConn1

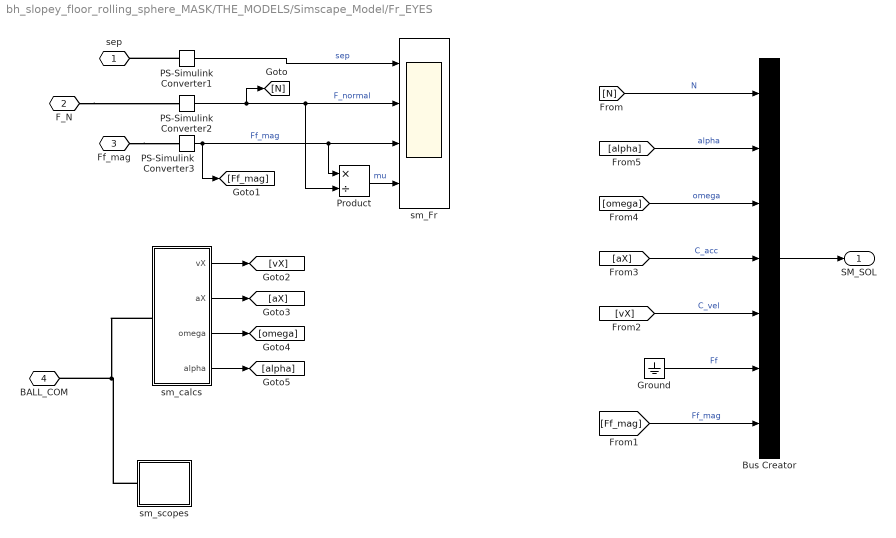
== system bh_slopey_floor_rolling_sphere_MASK/THE_MODELS/Simscape_Model/Fr_EYES ==
  Bus Creator : BusCreator  Inputs=7
  Ground : Ground
  PS-Simulink Converter1 : nesl_utility/PS-Simulink Converter  PhysicalDomain=network_engine_domain  SubClassName=ps_output  LeftPortType=input  RightPortType=output  PseudoPeriodic=off  Frequencies=[]  Unit=m  AffineConversion=off
  PS-Simulink Converter2 : nesl_utility/PS-Simulink Converter  PhysicalDomain=network_engine_domain  SubClassName=ps_output  LeftPortType=input  RightPortType=output  PseudoPeriodic=off  Frequencies=[]  Unit=N  AffineConversion=off
  PS-Simulink Converter3 : nesl_utility/PS-Simulink Converter  PhysicalDomain=network_engine_domain  SubClassName=ps_output  LeftPortType=input  RightPortType=output  PseudoPeriodic=off  Frequencies=[]  Unit=N  AffineConversion=off
  Product : Product  Inputs=*/
  sm_Fr : Scope  NumInputPorts=4
  sm_calcs : Subsystem
  sm_scopes : Subsystem
  sep : PMIOPort  Side=Left
  F_N : PMIOPort  Port=2  Side=Left
  Ff_mag : PMIOPort  Port=3  Side=Left
  BALL_COM : PMIOPort  Port=4  Side=Right
  SM_SOL : Outport
  wires:
  PS-Simulink Converter1/1 -> sm_Fr/1  "sep"
  PS-Simulink Converter2/1 -> [N], Product/2, sm_Fr/2  "F_normal"
  PS-Simulink Converter3/1 -> [Ff_mag], Product/1, sm_Fr/3  "Ff_mag"
  Bus Creator/1 -> SM_SOL/1
  [Ff_mag] -> Bus Creator/7  "Ff_mag"
  [omega] -> Bus Creator/3  "omega"
  [vX] -> Bus Creator/5  "C_vel"
  [alpha] -> Bus Creator/2  "alpha"
  [N] -> Bus Creator/1  "N"
  [aX] -> Bus Creator/4  "C_acc"
  Ground/1 -> Bus Creator/6  "Ff"
  sm_calcs/4(alpha) -> [alpha]
  sm_calcs/3(omega) -> [omega]
  sm_calcs/2(aX) -> [aX]
  sm_calcs/1(vX) -> [vX]
  Product/1 -> sm_Fr/4  "mu"
  connections:
  Ff_mag/RConn1 -- PS-Simulink Converter3/LConn1
  PS-Simulink Converter1/LConn1 -- sep/RConn1
  F_N/RConn1 -- PS-Simulink Converter2/LConn1
  sm_scopes/LConn1 -- sm_calcs/LConn1 -- BALL_COM/RConn1

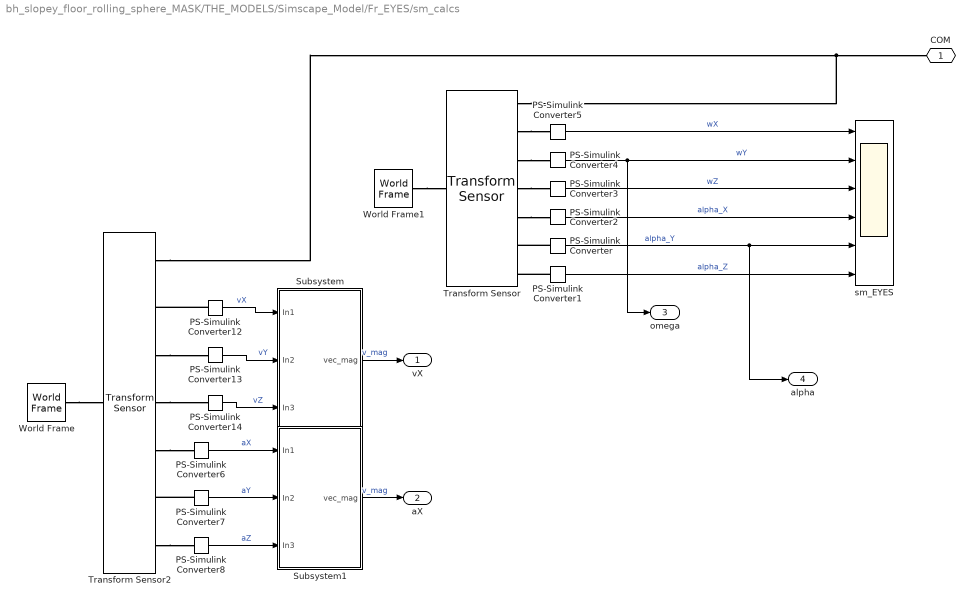
== system bh_slopey_floor_rolling_sphere_MASK/THE_MODELS/Simscape_Model/Fr_EYES/sm_calcs ==
  PS-Simulink Converter : nesl_utility/PS-Simulink Converter  PhysicalDomain=network_engine_domain  SubClassName=ps_output  LeftPortType=input  RightPortType=output  PseudoPeriodic=off  Frequencies=[]  Unit=rad/s^2  AffineConversion=off
  PS-Simulink Converter1 : nesl_utility/PS-Simulink Converter  PhysicalDomain=network_engine_domain  SubClassName=ps_output  LeftPortType=input  RightPortType=output  PseudoPeriodic=off  Frequencies=[]  Unit=rad/s^2  AffineConversion=off
  PS-Simulink Converter12 : nesl_utility/PS-Simulink Converter  PhysicalDomain=network_engine_domain  SubClassName=ps_output  LeftPortType=input  RightPortType=output  PseudoPeriodic=off  Frequencies=[]  Unit=m/s  AffineConversion=off
  PS-Simulink Converter13 : nesl_utility/PS-Simulink Converter  PhysicalDomain=network_engine_domain  SubClassName=ps_output  LeftPortType=input  RightPortType=output  PseudoPeriodic=off  Frequencies=[]  Unit=m/s  AffineConversion=off
  PS-Simulink Converter14 : nesl_utility/PS-Simulink Converter  PhysicalDomain=network_engine_domain  SubClassName=ps_output  LeftPortType=input  RightPortType=output  PseudoPeriodic=off  Frequencies=[]  Unit=m/s  AffineConversion=off
  PS-Simulink Converter2 : nesl_utility/PS-Simulink Converter  PhysicalDomain=network_engine_domain  SubClassName=ps_output  LeftPortType=input  RightPortType=output  PseudoPeriodic=off  Frequencies=[]  Unit=rad/s^2  AffineConversion=off
  PS-Simulink Converter3 : nesl_utility/PS-Simulink Converter  PhysicalDomain=network_engine_domain  SubClassName=ps_output  LeftPortType=input  RightPortType=output  PseudoPeriodic=off  Frequencies=[]  Unit=rad/s  AffineConversion=off
  PS-Simulink Converter4 : nesl_utility/PS-Simulink Converter  PhysicalDomain=network_engine_domain  SubClassName=ps_output  LeftPortType=input  RightPortType=output  PseudoPeriodic=off  Frequencies=[]  Unit=rad/s  AffineConversion=off
  PS-Simulink Converter5 : nesl_utility/PS-Simulink Converter  PhysicalDomain=network_engine_domain  SubClassName=ps_output  LeftPortType=input  RightPortType=output  PseudoPeriodic=off  Frequencies=[]  Unit=rad/s  AffineConversion=off
  PS-Simulink Converter6 : nesl_utility/PS-Simulink Converter  PhysicalDomain=network_engine_domain  SubClassName=ps_output  LeftPortType=input  RightPortType=output  PseudoPeriodic=off  Frequencies=[]  Unit=m/s^2  AffineConversion=off
  PS-Simulink Converter7 : nesl_utility/PS-Simulink Converter  PhysicalDomain=network_engine_domain  SubClassName=ps_output  LeftPortType=input  RightPortType=output  PseudoPeriodic=off  Frequencies=[]  Unit=m/s^2  AffineConversion=off
  PS-Simulink Converter8 : nesl_utility/PS-Simulink Converter  PhysicalDomain=network_engine_domain  SubClassName=ps_output  LeftPortType=input  RightPortType=output  PseudoPeriodic=off  Frequencies=[]  Unit=m/s^2  AffineConversion=off
  Subsystem : Subsystem
  Subsystem1 : Subsystem
  Transform Sensor : sm_lib/Frames and Transforms/Transform Sensor  MeasurementFrame=World  SenseAngle=off  SenseAxis=off  SenseAngle1=off  SenseAngle2=off  SenseAngle3=off  SenseQ=off  SenseR=off  SenseOmegaX=on  SenseOmegaY=on  SenseOmegaZ=on  SenseOmega1=off  SenseOmega2=off  SenseOmega3=off  SenseQDot=off  SenseRDot=off  SenseAlphaX=on  SenseAlphaY=on  SenseAlphaZ=on  SenseAlpha1=off  SenseAlpha2=off  SenseAlpha3=off  SenseQDDot=off  SenseRDDot=off  SenseX=off  SenseY=off  SenseZ=off  SenseRad=off  SenseAzim=off  SenseDist=off  SenseInc=off  SenseXDot=off  SenseYDot=off  SenseZDot=off  SenseRadDot=off  SenseAzimDot=off  SenseDistDot=off  SenseIncDot=off  SenseXDDot=off  SenseYDDot=off  SenseZDDot=off  SenseRadDDot=off  SenseAzimDDot=off  SenseDistDDot=off  SenseIncDDot=off
  Transform Sensor2 : sm_lib/Frames and Transforms/Transform Sensor  MeasurementFrame=World  SenseAngle=off  SenseAxis=off  SenseAngle1=off  SenseAngle2=off  SenseAngle3=off  SenseQ=off  SenseR=off  SenseOmegaX=off  SenseOmegaY=off  SenseOmegaZ=off  SenseOmega1=off  SenseOmega2=off  SenseOmega3=off  SenseQDot=off  SenseRDot=off  SenseAlphaX=off  SenseAlphaY=off  SenseAlphaZ=off  SenseAlpha1=off  SenseAlpha2=off  SenseAlpha3=off  SenseQDDot=off  SenseRDDot=off  SenseX=off  SenseY=off  SenseZ=off  SenseRad=off  SenseAzim=off  SenseDist=off  SenseInc=off  SenseXDot=on  SenseYDot=on  SenseZDot=on  SenseRadDot=off  SenseAzimDot=off  SenseDistDot=off  SenseIncDot=off  SenseXDDot=on  SenseYDDot=on  SenseZDDot=on  SenseRadDDot=off  SenseAzimDDot=off  SenseDistDDot=off  SenseIncDDot=off
  World Frame : sm_lib/Frames and Transforms/World Frame
  World Frame1 : sm_lib/Frames and Transforms/World Frame
  sm_EYES : Scope  NumInputPorts=6
  COM : PMIOPort  Side=Left
  vX : Outport
  aX : Outport  Port=2
  omega : Outport  Port=3
  alpha : Outport  Port=4
  wires:
  PS-Simulink Converter5/1 -> sm_EYES/1  "wX"
  PS-Simulink Converter4/1 -> sm_EYES/2, omega/1  "wY"
  PS-Simulink Converter3/1 -> sm_EYES/3  "wZ"
  PS-Simulink Converter/1 -> alpha/1, sm_EYES/5  "alpha_Y"
  PS-Simulink Converter1/1 -> sm_EYES/6  "alpha_Z"
  PS-Simulink Converter2/1 -> sm_EYES/4  "alpha_X"
  PS-Simulink Converter7/1 -> Subsystem1/2(In2)  "aY"
  PS-Simulink Converter6/1 -> Subsystem1/1(In1)  "aX"
  PS-Simulink Converter8/1 -> Subsystem1/3(In3)  "aZ"
  PS-Simulink Converter14/1 -> Subsystem/3(In3)  "vZ"
  PS-Simulink Converter13/1 -> Subsystem/2(In2)  "vY"
  PS-Simulink Converter12/1 -> Subsystem/1(In1)  "vX"
  Subsystem/1(vec_mag) -> vX/1  "v_mag"
  Subsystem1/1(vec_mag) -> aX/1  "v_mag"
  connections:
  Transform Sensor/RConn1 -- Transform Sensor2/RConn1 -- COM/RConn1
  PS-Simulink Converter1/LConn1 -- Transform Sensor/RConn7
  PS-Simulink Converter/LConn1 -- Transform Sensor/RConn6
  Transform Sensor/RConn5 -- PS-Simulink Converter2/LConn1
  Transform Sensor/RConn4 -- PS-Simulink Converter3/LConn1
  Transform Sensor/RConn3 -- PS-Simulink Converter4/LConn1
  Transform Sensor/RConn2 -- PS-Simulink Converter5/LConn1
  PS-Simulink Converter12/LConn1 -- Transform Sensor2/RConn2
  Transform Sensor2/RConn4 -- PS-Simulink Converter14/LConn1
  Transform Sensor2/RConn3 -- PS-Simulink Converter13/LConn1
  World Frame/RConn1 -- Transform Sensor2/LConn1
  World Frame1/RConn1 -- Transform Sensor/LConn1
  Transform Sensor2/RConn5 -- PS-Simulink Converter6/LConn1
  PS-Simulink Converter7/LConn1 -- Transform Sensor2/RConn6
  Transform Sensor2/RConn7 -- PS-Simulink Converter8/LConn1

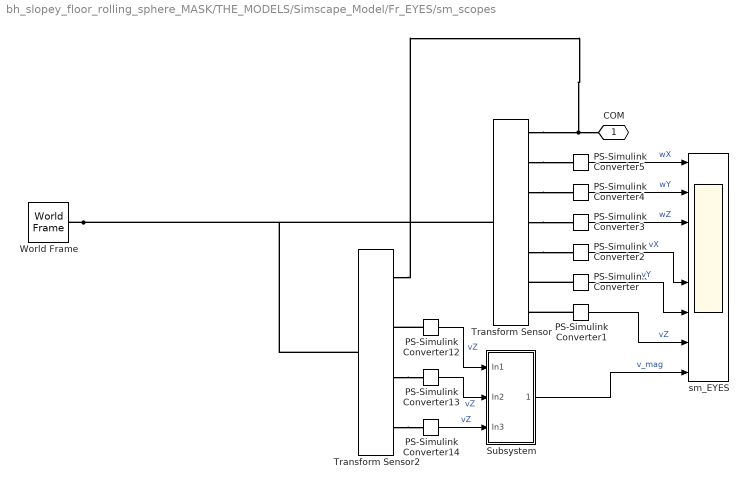
== system bh_slopey_floor_rolling_sphere_MASK/THE_MODELS/Simscape_Model/Fr_EYES/sm_scopes ==
  PS-Simulink Converter{,1..2,12..14} (6 alike) : nesl_utility/PS-Simulink Converter  PhysicalDomain=network_engine_domain  SubClassName=ps_output  LeftPortType=input  RightPortType=output  PseudoPeriodic=off  Frequencies=[]  Unit=m/s  AffineConversion=off
  PS-Simulink Converter3 : nesl_utility/PS-Simulink Converter  PhysicalDomain=network_engine_domain  SubClassName=ps_output  LeftPortType=input  RightPortType=output  PseudoPeriodic=off  Frequencies=[]  Unit=rad/s  AffineConversion=off
  PS-Simulink Converter4 : nesl_utility/PS-Simulink Converter  PhysicalDomain=network_engine_domain  SubClassName=ps_output  LeftPortType=input  RightPortType=output  PseudoPeriodic=off  Frequencies=[]  Unit=rad/s  AffineConversion=off
  PS-Simulink Converter5 : nesl_utility/PS-Simulink Converter  PhysicalDomain=network_engine_domain  SubClassName=ps_output  LeftPortType=input  RightPortType=output  PseudoPeriodic=off  Frequencies=[]  Unit=rad/s  AffineConversion=off
  Subsystem : Subsystem
  Transform Sensor : sm_lib/Frames and Transforms/Transform Sensor  MeasurementFrame=World  SenseAngle=off  SenseAxis=off  SenseAngle1=off  SenseAngle2=off  SenseAngle3=off  SenseQ=off  SenseR=off  SenseOmegaX=on  SenseOmegaY=on  SenseOmegaZ=on  SenseOmega1=off  SenseOmega2=off  SenseOmega3=off  SenseQDot=off  SenseRDot=off  SenseAlphaX=off  SenseAlphaY=off  SenseAlphaZ=off  SenseAlpha1=off  SenseAlpha2=off  SenseAlpha3=off  SenseQDDot=off  SenseRDDot=off  SenseX=off  SenseY=off  SenseZ=off  SenseRad=off  SenseAzim=off  SenseDist=off  SenseInc=off  SenseXDot=on  SenseYDot=on  SenseZDot=on  SenseRadDot=off  SenseAzimDot=off  SenseDistDot=off  SenseIncDot=off  SenseXDDot=off  SenseYDDot=off  SenseZDDot=off  SenseRadDDot=off  SenseAzimDDot=off  SenseDistDDot=off  SenseIncDDot=off
  Transform Sensor2 : sm_lib/Frames and Transforms/Transform Sensor  MeasurementFrame=World  SenseAngle=off  SenseAxis=off  SenseAngle1=off  SenseAngle2=off  SenseAngle3=off  SenseQ=off  SenseR=off  SenseOmegaX=off  SenseOmegaY=off  SenseOmegaZ=off  SenseOmega1=off  SenseOmega2=off  SenseOmega3=off  SenseQDot=off  SenseRDot=off  SenseAlphaX=off  SenseAlphaY=off  SenseAlphaZ=off  SenseAlpha1=off  SenseAlpha2=off  SenseAlpha3=off  SenseQDDot=off  SenseRDDot=off  SenseX=off  SenseY=off  SenseZ=off  SenseRad=off  SenseAzim=off  SenseDist=off  SenseInc=off  SenseXDot=on  SenseYDot=on  SenseZDot=on  SenseRadDot=off  SenseAzimDot=off  SenseDistDot=off  SenseIncDot=off  SenseXDDot=off  SenseYDDot=off  SenseZDDot=off  SenseRadDDot=off  SenseAzimDDot=off  SenseDistDDot=off  SenseIncDDot=off
  World Frame : sm_lib/Frames and Transforms/World Frame
  sm_EYES : Scope  NumInputPorts=8
  COM : PMIOPort  Side=Left
  wires:
  PS-Simulink Converter5/1 -> sm_EYES/1  "wX"
  PS-Simulink Converter4/1 -> sm_EYES/2  "wY"
  PS-Simulink Converter3/1 -> sm_EYES/3  "wZ"
  PS-Simulink Converter/1 -> sm_EYES/6  "vY"
  PS-Simulink Converter1/1 -> sm_EYES/7  "vZ"
  PS-Simulink Converter2/1 -> sm_EYES/5  "vX"
  Subsystem/1(v_mag) -> sm_EYES/8  "v_mag"
  PS-Simulink Converter12/1 -> Subsystem/1(In1)  "vZ"
  PS-Simulink Converter14/1 -> Subsystem/3(In3)  "vZ"
  PS-Simulink Converter13/1 -> Subsystem/2(In2)  "vZ"
  connections:
  World Frame/RConn1 -- Transform Sensor/LConn1 -- Transform Sensor2/LConn1
  Transform Sensor/RConn1 -- Transform Sensor2/RConn1 -- COM/RConn1
  PS-Simulink Converter1/LConn1 -- Transform Sensor/RConn7
  PS-Simulink Converter/LConn1 -- Transform Sensor/RConn6
  Transform Sensor/RConn5 -- PS-Simulink Converter2/LConn1
  Transform Sensor/RConn4 -- PS-Simulink Converter3/LConn1
  Transform Sensor/RConn3 -- PS-Simulink Converter4/LConn1
  Transform Sensor/RConn2 -- PS-Simulink Converter5/LConn1
  PS-Simulink Converter12/LConn1 -- Transform Sensor2/RConn2
  Transform Sensor2/RConn4 -- PS-Simulink Converter14/LConn1
  Transform Sensor2/RConn3 -- PS-Simulink Converter13/LConn1

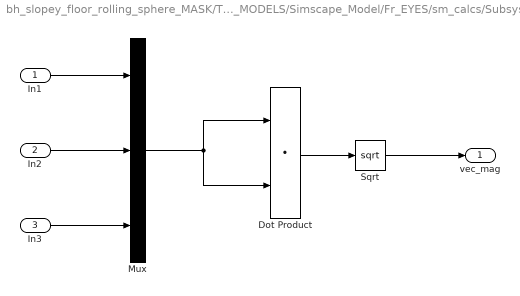
== system bh_slopey_floor_rolling_sphere_MASK/THE_MODELS/Simscape_Model/Fr_EYES/sm_calcs/Subsystem ==
  In1 : Inport
  In2 : Inport  Port=2
  In3 : Inport  Port=3
  Dot Product : DotProduct  InputSameDT=on  OutDataTypeStr=Inherit: Inherit via internal rule
  Mux : Mux  Inputs=3
  Sqrt : Sqrt  SaturateOnIntegerOverflow=on
  vec_mag : Outport
  wires:
  In2/1 -> Mux/2
  In1/1 -> Mux/1
  In3/1 -> Mux/3
  Mux/1 -> Dot Product/2, Dot Product/1
  Dot Product/1 -> Sqrt/1
  Sqrt/1 -> vec_mag/1

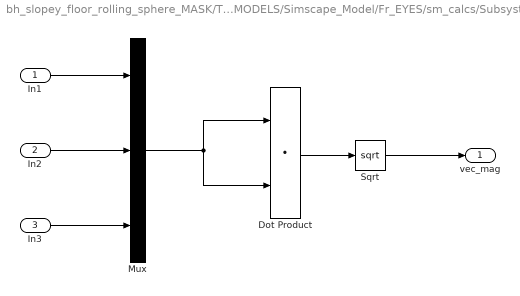
== system bh_slopey_floor_rolling_sphere_MASK/THE_MODELS/Simscape_Model/Fr_EYES/sm_calcs/Subsystem1 ==
  In1 : Inport
  In2 : Inport  Port=2
  In3 : Inport  Port=3
  Dot Product : DotProduct  InputSameDT=on  OutDataTypeStr=Inherit: Inherit via internal rule
  Mux : Mux  Inputs=3
  Sqrt : Sqrt  SaturateOnIntegerOverflow=on
  vec_mag : Outport
  wires:
  In2/1 -> Mux/2
  In1/1 -> Mux/1
  In3/1 -> Mux/3
  Mux/1 -> Dot Product/2, Dot Product/1
  Dot Product/1 -> Sqrt/1
  Sqrt/1 -> vec_mag/1

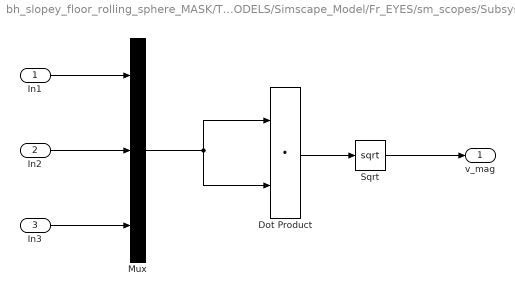
== system bh_slopey_floor_rolling_sphere_MASK/THE_MODELS/Simscape_Model/Fr_EYES/sm_scopes/Subsystem ==
  In1 : Inport
  In2 : Inport  Port=2
  In3 : Inport  Port=3
  Dot Product : DotProduct  InputSameDT=on  OutDataTypeStr=Inherit: Inherit via internal rule
  Mux : Mux  Inputs=3
  Sqrt : Sqrt  SaturateOnIntegerOverflow=on
  v_mag : Outport
  wires:
  In2/1 -> Mux/2
  In1/1 -> Mux/1
  In3/1 -> Mux/3
  Mux/1 -> Dot Product/2, Dot Product/1
  Dot Product/1 -> Sqrt/1
  Sqrt/1 -> v_mag/1
